simulink model "force_elements"  (R2021a)
settings: Solver=VariableStepAuto  StartTime=0.0  StopTime=10.0  RelTol=1e-3
settings Model: Creator=jadg1  LastModifiedBy=jadg1

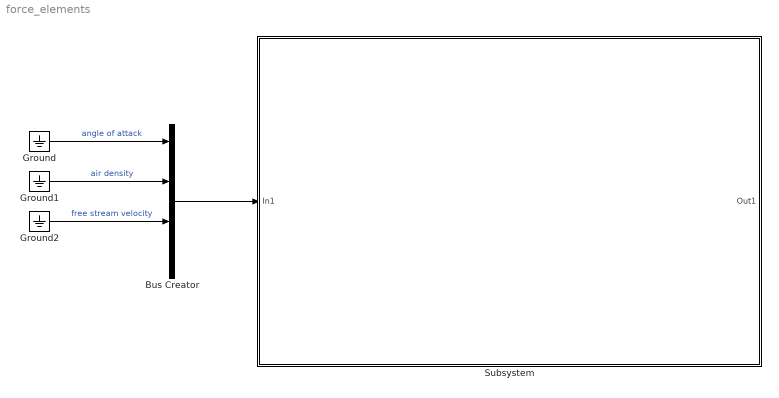
== system force_elements ==
  Bus Creator : BusCreator  Inputs=4
  Ground : Ground
  Ground1 : Ground
  Ground2 : Ground
  Subsystem : Subsystem
  wires:
  Bus Creator/1 -> Subsystem/1(In1)
  Ground/1 -> Bus Creator/1  "angle of attack"
  Ground1/1 -> Bus Creator/2  "air density"
  Ground2/1 -> Bus Creator/3  "free stream velocity"
  ? -> Bus Creator/4

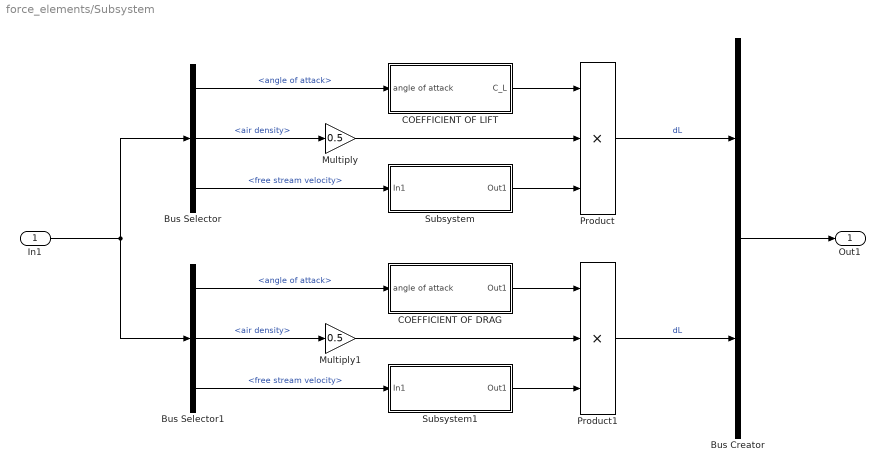
== system force_elements/Subsystem ==
  In1 : Inport
  Bus Creator : BusCreator  Inputs=2
  Bus Selector : BusSelector  OutputSignals=angle of attack,air density,free stream velocity
  Bus Selector1 : BusSelector  OutputSignals=angle of attack,air density,free stream velocity
  COEFFICIENT OF DRAG : Subsystem
  "COEFFICIENT OF LIFT " : Subsystem
  Multiply : Gain  Gain=0.5
  Multiply1 : Gain  Gain=0.5
  Product : Product  Inputs=3
  Product1 : Product  Inputs=3
  Subsystem : Subsystem
  Subsystem1 : Subsystem
  Out1 : Outport
  wires:
  In1/1 -> Bus Selector/1, Bus Selector1/1
  Bus Selector/1 -> "COEFFICIENT OF LIFT "/1(angle of attack)  "<angle of attack>"
  Bus Selector/2 -> Multiply/1  "<air density>"
  Bus Selector/3 -> Subsystem/1(In1)  "<free stream velocity>"
  Multiply/1 -> Product/2
  "COEFFICIENT OF LIFT "/1(C_L) -> Product/1
  Subsystem/1(Out1) -> Product/3
  Product/1 -> Bus Creator/1  "dL"
  Bus Creator/1 -> Out1/1
  Bus Selector1/1 -> COEFFICIENT OF DRAG/1(angle of attack)  "<angle of attack>"
  Product1/1 -> Bus Creator/2  "dL"
  Subsystem1/1(Out1) -> Product1/3
  Multiply1/1 -> Product1/2
  Bus Selector1/3 -> Subsystem1/1(In1)  "<free stream velocity>"
  Bus Selector1/2 -> Multiply1/1  "<air density>"
  COEFFICIENT OF DRAG/1(Out1) -> Product1/1

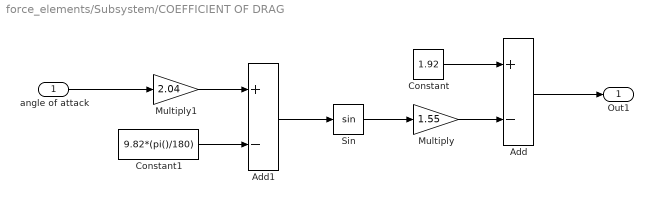
== system force_elements/Subsystem/COEFFICIENT OF DRAG ==
  angle of attack : Inport
  Add : Sum  Inputs=+-
  Add1 : Sum  Inputs=+-
  Constant : Constant  Value=1.92
  Constant1 : Constant  Value=9.82*(pi()/180)
  Multiply : Gain  Gain=1.55
  Multiply1 : Gain  Gain=2.04
  Sin : Trigonometry
  Out1 : Outport
  wires:
  Multiply1/1 -> Add1/1
  Multiply/1 -> Add/2
  Add1/1 -> Sin/1
  Constant/1 -> Add/1
  Add/1 -> Out1/1
  angle of attack/1 -> Multiply1/1
  Sin/1 -> Multiply/1
  Constant1/1 -> Add1/2

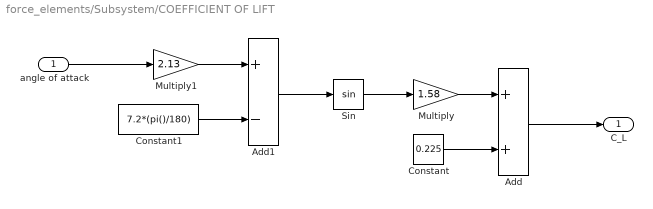
== system force_elements/Subsystem/COEFFICIENT OF LIFT  ==
  angle of attack : Inport
  Add : Sum
  Add1 : Sum  Inputs=+-
  Constant : Constant  Value=0.225
  Constant1 : Constant  Value=7.2*(pi()/180)
  Multiply : Gain  Gain=1.58
  Multiply1 : Gain  Gain=2.13
  Sin : Trigonometry
  C_L : Outport
  wires:
  Add/1 -> C_L/1
  Constant/1 -> Add/2
  Multiply/1 -> Add/1
  Sin/1 -> Multiply/1
  Add1/1 -> Sin/1
  angle of attack/1 -> Multiply1/1
  Multiply1/1 -> Add1/1
  Constant1/1 -> Add1/2

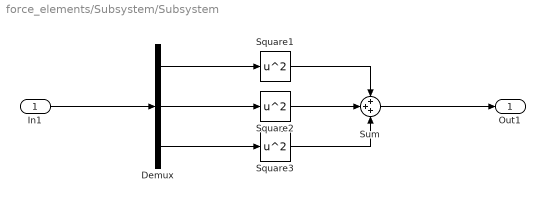
== system force_elements/Subsystem/Subsystem ==
  In1 : Inport
  Demux : Demux  Outputs=3
  Square1 : Math  Operator=square  SaturateOnIntegerOverflow=on
  Square2 : Math  Operator=square  SaturateOnIntegerOverflow=on
  Square3 : Math  Operator=square  SaturateOnIntegerOverflow=on
  Sum : Sum  Inputs=+++
  Out1 : Outport
  wires:
  Square2/1 -> Sum/2
  Square3/1 -> Sum/3
  Square1/1 -> Sum/1
  Sum/1 -> Out1/1
  In1/1 -> Demux/1
  Demux/1 -> Square1/1
  Demux/2 -> Square2/1
  Demux/3 -> Square3/1

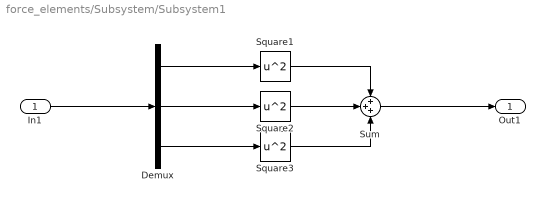
== system force_elements/Subsystem/Subsystem1 ==
  In1 : Inport
  Demux : Demux  Outputs=3
  Square1 : Math  Operator=square  SaturateOnIntegerOverflow=on
  Square2 : Math  Operator=square  SaturateOnIntegerOverflow=on
  Square3 : Math  Operator=square  SaturateOnIntegerOverflow=on
  Sum : Sum  Inputs=+++
  Out1 : Outport
  wires:
  Demux/3 -> Square3/1
  Demux/2 -> Square2/1
  Demux/1 -> Square1/1
  In1/1 -> Demux/1
  Sum/1 -> Out1/1
  Square1/1 -> Sum/1
  Square3/1 -> Sum/3
  Square2/1 -> Sum/2
